simulink model "BusSelector4"  (R2017b)
settings: Solver=FixedStepDiscrete  StartTime=0.0  StopTime=10.0  RelTol=1e-3  EnableMultiTasking=on
PreLoadFcn:
  | busCell = { ...
  |         { ...
  |             'InputBus', ...
  |             'MyHeader.h', ...
  |             'My description', ...
  |             'Exported', ...
  |             '-1', ...
  |             {{'enable',1,'double', [0.2 0],'real','Sample'}; ...
  |              {'brake',1,'double', [0.2 0],'real','Sample'}; ...
  |              {'Actual_speed',1,'double', [0.2 0],'real','Sample'}; ...
  |              {'set',1,'double', [0.2 0],'real','Sample'}; ...
  |             {'inc',1,'double', [0.2 0],'real','Sample'}; ...
  |             {'dec',1,'double', [0.2 0],'real','Sample'}},...
  |             }, ...
  |         };
  | Simulink.Bus.cellToObject(busCell)
model workspace (MAT data in the model file):
  C = {{'InputBus', '', '', 'Auto', '-1', {{'Actual_speed', 1, 'double', -1, 'real', 'Sample', 'Fixed', [], [], '', ''}; {'Switches', 1, 'Switches', -1, 'real', 'Sample', 'Fixed', [], [], '', ''}}}; {'InputBusFxp', '', '', 'Auto', '-1', {{'Actual_speed', 1, 'fixdt(0,16,8)', -1, 'real', 'Sample', 'Fixed', [], [], '', ''}; {'Switches', 1, 'Switches', -1, 'real', 'Sample', 'Fixed', [], [], '', ''}}}; {'Switches', '', '', 'Auto', '-1', {{'enable', 1, 'boolean', -1, 'real', 'Sample', 'Fixed', [], [], '', ''}; {'brake', 1, 'boolean', -1, 'real', 'Sample', 'Fixed', [], [], '', ''}; {'set', 1, 'boolean', -1, 'real', 'Sample', 'Fixed', [], [], '', ''}; {'setIncDec', 1, 'setpoint', -1, 'real', 'Sample', 'Fixed', [], [], '', ''}}}; {'ccOut', '', '', 'Auto', '-1', {{'reqDrv', 1, 'Enum: reqMode', -1, 'real', 'Sample', 'Fixed', [], [], '', ''}; {'status', 1, 'boolean', -1, 'real', 'Sample', 'Fixed', [], [], '', ''}; {'mode', 1, 'Enum: opMode', -1, 'real', 'Sample', 'Fixed', [], [], '', ''}; {'targetSp', 1, 'double', -1, 'real', 'Sample', 'Fixed', [], [], '', ''}; {'throtCC', 1, 'double', -1, 'real', 'Sample', 'Fixed', [], [], '', ''}}}; {'sbrInputs', '', '', 'Auto', '-1', {{'Speed', 1, 'fixdt(0,16,2)', -1, 'real', 'Sample', 'Fixed', [], [], '', ''}; {'SeatBeltFasten', 1, 'boolean', -1, 'real', 'Sample', 'Fixed', [], [], '', ''}; {'KEY', 1, 'int8', -1, 'real', 'Sample', 'Fixed', [], [], '', ''}}}; {'setpoint', '', '', 'Auto', '-1', {{'inc', 1, 'boolean', -1, 'real', 'Sample', 'Fixed', [], [], '', ''}; {'dec', 1, 'boolean', -1, 'real', 'Sample', 'Fixed', [], [], '', ''}}}; {'sldvThrustReverseBus', '', '', 'Auto', '-1', {{'wowSensors', 4, 'boolean', -1, 'real', 'Sample', 'Fixed', [], [], '', ''}; {'wheelSpeedSensors', 2, 'double', -1, 'real', 'Sample', 'Fixed', [], [], '', ''}; {'airSpeedSensors', 2, 'double', -1, 'real', 'Sample', 'Fixed', [], [], '', ''}; {'throttlePositions', 4, 'double', -1, 'real', 'Sample', 'Fixed', [], [], '', ''}}}}
settings Model: Creator=hbourbou  LastModifiedBy=hbourbou
settings OptimizationCC: LifeSpan=inf
settings DebuggingCC: SFExecutionAtInitializationDiag=none
settings HardwareCC: ProdBitPerSizeT=32  ProdBitPerPtrDiffT=32  ProdWordSize=32  ProdHWDeviceType=Specified
settings CodeAppCC: StateflowObjectComments=on

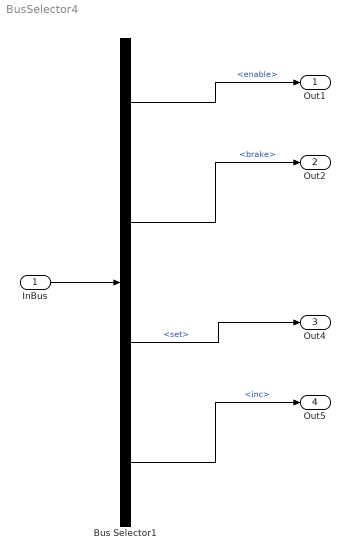
== system BusSelector4 ==
  InBus : Inport  OutDataTypeStr=Bus: InputBus  PortDimensions=1  BusOutputAsStruct=on
  Bus Selector1 : BusSelector  OutputSignals=enable,brake,set,inc
  Out1 : Outport
  Out2 : Outport  Port=2
  Out4 : Outport  Port=3
  Out5 : Outport  Port=4
  wires:
  InBus/1 -> Bus Selector1/1
  Bus Selector1/3 -> Out4/1  "<set>"
  Bus Selector1/1 -> Out1/1  "<enable>"
  Bus Selector1/2 -> Out2/1  "<brake>"
  Bus Selector1/4 -> Out5/1  "<inc>"
